simulink model "Simulink_ROS_Boat_Path_Follow_V2_5"  (R2025b)
settings: Solver=FixedStepAuto  StartTime=0.0  StopTime=2500  FixedStep=0.001  RelTol=1e-3
undefined symbols (not defined in the file): init_psi, init_x, init_y, path_x, path_y
libraries: ros2lib x6, slpidlib x2
settings Model: NumberOfSteps=10  Creator=Semih  LastModifiedBy=gehan
settings SolverCC: EnableFixedStepZeroCrossing=on

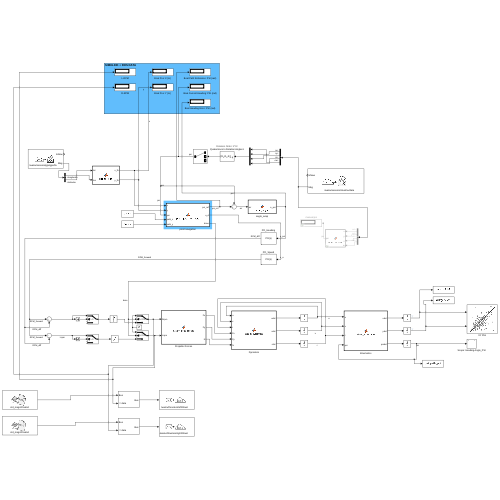
[thumbnail: Simulink's stored preview of the top-level diagram]
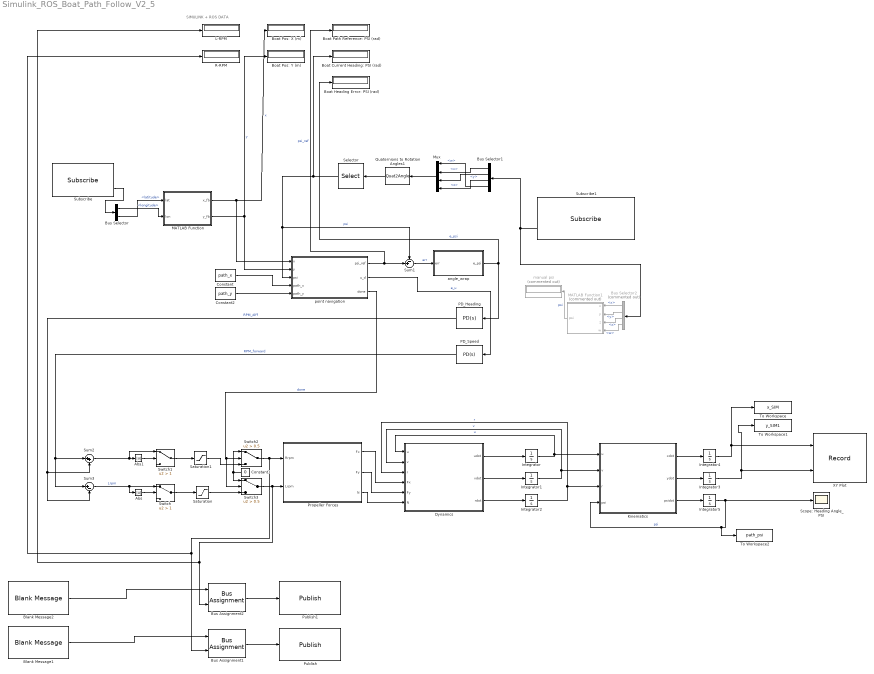
== system Simulink_ROS_Boat_Path_Follow_V2_5 ==
  note: SIMULINK + ROS DATA
  Abs : Abs  SaturateOnIntegerOverflow=off
  Abs1 : Abs  SaturateOnIntegerOverflow=off
  Blank Message1 : ros2lib/Blank Message  messageClass=Message  entityType=std_msgs/Float64  messageType=std_msgs/Float64  SampleTime=inf
  Blank Message2 : ros2lib/Blank Message  messageClass=Message  entityType=std_msgs/Float64  messageType=std_msgs/Float64  SampleTime=inf
  Boat Current Heading: PSI (rad) : Display
  Boat Heading Error: PSI (rad) : Display
  Boat Path Reference: PSI (rad) : Display
  Boat Pos: X (m) : Display
  Boat Pos: Y (m) : Display
  Bus Assignment1 : BusAssignment  AssignedSignals=data
  Bus Assignment2 : BusAssignment  AssignedSignals=data
  Bus Selector : BusSelector  OutputSignals=longitude,latitude
  Bus Selector1 : BusSelector  OutputSignals=orientation.x,orientation.y,orientation.z,orientation.w
  Bus Selector2 : BusSelector  Commented=on  OutputSignals=orientation.x,orientation.y,orientation.z,orientation.w
  Constant : Constant  Value=path_x
  Constant1 : Constant  Value=0
  Constant2 : Constant  Value=path_y
  Dynamics : MATLAB Function  TreatAsAtomicUnit=on
  Integrator : Integrator
  Integrator1 : Integrator
  Integrator2 : Integrator
  Integrator3 : Integrator  InitialCondition=init_y
  Integrator4 : Integrator  InitialCondition=init_x
  Integrator5 : Integrator  InitialCondition=init_psi
  Kinematics : MATLAB Function  TreatAsAtomicUnit=on
  L-RPM : Display
  MATLAB Function : MATLAB Function  TreatAsAtomicUnit=on
  MATLAB Function1 : MATLAB Function  Commented=on  TreatAsAtomicUnit=on
  Mux : Mux
  PD_Heading : slpidlib/PID Controller  Controller=PD  Form=Parallel  TimeDomain=Continuous-time  UseExternalTs=off  SampleTime=-1  IntegratorMethod=Forward Euler  FilterMethod=Forward Euler  ControllerParametersSource=internal  P=200  I=0  UseKiTs=off  D=5  UseExternalDerivativeSource=off  N=50  UseFilter=on  TunerSelectOption=Transfer Function Based (PID Tuner App)  InitialConditionSource=internal  InitialConditionForIntegrator=0  InitialConditionForFilter=0  DifferentiatorICPrevScaledInput=0  ExternalReset=none  TrackingMode=off  Kt=1  LimitOutput=off  SatLimitsSource=internal  UpperSaturationLimit=300  LowerSaturationLimit=-300  LinearizeAsGain=on  AntiWindupMode=back-calculation  Kb=1  LimitIntegrator=off  UpperIntegratorSaturationLimit=inf  LowerIntegratorSaturationLimit=-inf  POutMin=[]  POutMax=[]  IOutMin=[]  IOutMax=[]  DOutMin=[]  DOutMax=[]  NOutMin=[]  NOutMax=[]  SumOutMin=[]  SumOutMax=[]  SaturationOutMin=[]  SaturationOutMax=[]  PParamMin=[]  PParamMax=[]  IParamMin=[]  IParamMax=[]  DParamMin=[]  DParamMax=[]  NParamMin=[]  NParamMax=[]  KbParamMin=[]  KbParamMax=[]  KtParamMin=[]  KtParamMax=[]  KbOutMin=[]  KbOutMax=[]  KtOutMin=[]  KtOutMax=[]  IntegratorOutMin=[]  IntegratorOutMax=[]  FilterOutMin=[]  FilterOutMax=[]  SumI1OutMin=[]  SumI1OutMax=[]  SumI2OutMin=[]  SumI2OutMax=[]  SumI3OutMin=[]  SumI3OutMax=[]  SumI4OutMin=[]  SumI4OutMax=[]  SumDOutMin=[]  SumDOutMax=[]  DifferentiatorOutMin=[]  DifferentiatorOutMax=[]  FilterDiffOutCoefMin=[]  FilterDiffOutCoefMax=[]  ReciprocalOutMin=[]  ReciprocalOutMax=[]  SumDenOutMin=[]  SumDenOutMax=[]  SumNumOutMin=[]  SumNumOutMax=[]  DivideOutMin=[]  DivideOutMax=[]  UdiffTsProdOutMin=[]  UdiffTsProdOutMax=[]  NTsProdOutMin=[]  NTsProdOutMax=[]  UintegralTsProdOutMin=[]  UintegralTsProdOutMax=[]  UngainTsProdOutMin=[]  UngainTsProdOutMax=[]  ClampingZeroOutDataTypeStr=Inherit: Inherit via back propagation  ClampingZeroOutMin=[]  ClampingZeroOutMax=[]  FilterDenConstantOutDataTypeStr=Inherit: Inherit via back propagation  FilterDenConstantOutMin=[]  FilterDenConstantOutMax=[]  PCopyOutDataTypeStr=Inherit: Inherit via back propagation  PCopyOutMin=[]  PCopyOutMax=[]  NCopyOutDataTypeStr=Inherit: Inherit via back propagation  NCopyOutMin=[]  NCopyOutMax=[]  IntegratorContinuousStateAttributes=''  IntegratorStateMustResolveToSignalObject=off  IntegratorRTWStateStorageClass=Auto  FilterContinuousStateAttributes=''  FilterStateMustResolveToSignalObject=off  FilterRTWStateStorageClass=Auto  ParallelPVariant=InternalParameters  IdealPVariant=Disabled  IVariant=Disabled  DVariant=InternalParameters  IntegratorVariant=Disabled  SatVariant=Disabled  AWVariant=Disabled  PCopyVariant=Disabled  TRVariant=Disabled  FdbkBlocksVariant=Forward  IdealPFdbkVariant=Disabled  SatFdbkVariant=Disabled  DerivativeFilterVariant=ContFilter  NVariant=InternalParameters  NCopyVariant=Disabled  FilterICVariant=InternalICsFilter  IntegratorICVariant=Disabled  ExternalResetVariant=Disabled  TRSumVariant=Passthrough  SumFdbkVariant=Disabled  SumVariant=Sum_PD  TsampFilterVariant=InternalTs  TsampNgainVariant=Passthrough  TsampIntegralVariant=Disabled_SignalSpec  ExternalSaturationOutDataTypeStr=Inherit: Same as second input  DerivativeSourceVariant=ErrorSignal  PreIntVariant=InternalPreInt
  PD_Speed : slpidlib/PID Controller  Controller=PD  Form=Parallel  TimeDomain=Continuous-time  UseExternalTs=off  SampleTime=-1  IntegratorMethod=Forward Euler  FilterMethod=Forward Euler  ControllerParametersSource=internal  P=100  I=5  UseKiTs=off  D=5  UseExternalDerivativeSource=off  N=50  UseFilter=on  TunerSelectOption=Transfer Function Based (PID Tuner App)  InitialConditionSource=internal  InitialConditionForIntegrator=0  InitialConditionForFilter=0  DifferentiatorICPrevScaledInput=0  ExternalReset=none  TrackingMode=off  Kt=1  LimitOutput=off  SatLimitsSource=internal  UpperSaturationLimit=inf  LowerSaturationLimit=-inf  LinearizeAsGain=on  AntiWindupMode=none  Kb=1  LimitIntegrator=off  UpperIntegratorSaturationLimit=inf  LowerIntegratorSaturationLimit=-inf  POutMin=[]  POutMax=[]  IOutMin=[]  IOutMax=[]  DOutMin=[]  DOutMax=[]  NOutMin=[]  NOutMax=[]  SumOutMin=[]  SumOutMax=[]  SaturationOutMin=[]  SaturationOutMax=[]  PParamMin=[]  PParamMax=[]  IParamMin=[]  IParamMax=[]  DParamMin=[]  DParamMax=[]  NParamMin=[]  NParamMax=[]  KbParamMin=[]  KbParamMax=[]  KtParamMin=[]  KtParamMax=[]  KbOutMin=[]  KbOutMax=[]  KtOutMin=[]  KtOutMax=[]  IntegratorOutMin=[]  IntegratorOutMax=[]  FilterOutMin=[]  FilterOutMax=[]  SumI1OutMin=[]  SumI1OutMax=[]  SumI2OutMin=[]  SumI2OutMax=[]  SumI3OutMin=[]  SumI3OutMax=[]  SumI4OutMin=[]  SumI4OutMax=[]  SumDOutMin=[]  SumDOutMax=[]  DifferentiatorOutMin=[]  DifferentiatorOutMax=[]  FilterDiffOutCoefMin=[]  FilterDiffOutCoefMax=[]  ReciprocalOutMin=[]  ReciprocalOutMax=[]  SumDenOutMin=[]  SumDenOutMax=[]  SumNumOutMin=[]  SumNumOutMax=[]  DivideOutMin=[]  DivideOutMax=[]  UdiffTsProdOutMin=[]  UdiffTsProdOutMax=[]  NTsProdOutMin=[]  NTsProdOutMax=[]  UintegralTsProdOutMin=[]  UintegralTsProdOutMax=[]  UngainTsProdOutMin=[]  UngainTsProdOutMax=[]  ClampingZeroOutDataTypeStr=Inherit: Inherit via back propagation  ClampingZeroOutMin=[]  ClampingZeroOutMax=[]  FilterDenConstantOutDataTypeStr=Inherit: Inherit via back propagation  FilterDenConstantOutMin=[]  FilterDenConstantOutMax=[]  PCopyOutDataTypeStr=Inherit: Inherit via back propagation  PCopyOutMin=[]  PCopyOutMax=[]  NCopyOutDataTypeStr=Inherit: Inherit via back propagation  NCopyOutMin=[]  NCopyOutMax=[]  IntegratorContinuousStateAttributes=''  IntegratorStateMustResolveToSignalObject=off  IntegratorRTWStateStorageClass=Auto  FilterContinuousStateAttributes=''  FilterStateMustResolveToSignalObject=off  FilterRTWStateStorageClass=Auto  ParallelPVariant=InternalParameters  IdealPVariant=Disabled  IVariant=Disabled  DVariant=InternalParameters  IntegratorVariant=Disabled  SatVariant=Disabled  AWVariant=Disabled  PCopyVariant=Disabled  TRVariant=Disabled  FdbkBlocksVariant=Forward  IdealPFdbkVariant=Disabled  SatFdbkVariant=Disabled  DerivativeFilterVariant=ContFilter  NVariant=InternalParameters  NCopyVariant=Disabled  FilterICVariant=InternalICsFilter  IntegratorICVariant=Disabled  ExternalResetVariant=Disabled  TRSumVariant=Passthrough  SumFdbkVariant=Disabled  SumVariant=Sum_PD  TsampFilterVariant=InternalTs  TsampNgainVariant=Passthrough  TsampIntegralVariant=Disabled_SignalSpec  ExternalSaturationOutDataTypeStr=Inherit: Same as second input  DerivativeSourceVariant=ErrorSignal  PreIntVariant=InternalPreInt
  Propeller Forces : MATLAB Function  TreatAsAtomicUnit=on
  Publish : ros2lib/Publish  topicSource=Specify your own  topic=/wamv/thrusters/right/thrust  messageType=std_msgs/Float64  QOSHistory=Keep last  QOSDepth=10  QOSReliability=Reliable  QOSDurability=Volatile  QOSDeadline=Inf  QOSLifespan=Inf  QOSLiveliness=Automatic  QOSLeaseDuration=Inf  QOSAvoidROSNamespaceConventions=off
  Publish1 : ros2lib/Publish  topicSource=Specify your own  topic=/wamv/thrusters/left/thrust  messageType=std_msgs/Float64  QOSHistory=Keep last  QOSDepth=10  QOSReliability=Reliable  QOSDurability=Volatile  QOSDeadline=Inf  QOSLifespan=Inf  QOSLiveliness=Automatic  QOSLeaseDuration=Inf  QOSAvoidROSNamespaceConventions=off
  Quaternions to Rotation Angles1 : Quat2Angle
      settings: AttributesFormatString=Rotation Order: %<rotationOrder>
  R-RPM : Display
  Saturation : Saturate  UpperLimit=1000  LowerLimit=0
  Saturation1 : Saturate  UpperLimit=1000  LowerLimit=0
  Scope: Heading Angle_PSI : Scope
      settings: ActiveDisplayYMinimum=-6.15148375375635  ActiveDisplayYMaximum=4.7778710179272776
  Selector : Selector  InputPortWidth=3  IndexOptions=Index vector (dialog)  Indices=1  OutputSizes=1
  Subscribe : ros2lib/Subscribe  topicSource=Specify your own  topic=/wamv/sensors/gps/gps/fix  messageType=sensor_msgs/NavSatFix  sampleTime=-1  QOSHistory=Keep last  QOSDepth=10  QOSReliability=Reliable  QOSDurability=Volatile  QOSDeadline=Inf  QOSLifespan=Inf  QOSLiveliness=Automatic  QOSLeaseDuration=Inf  QOSAvoidROSNamespaceConventions=off
  Subscribe1 : ros2lib/Subscribe  topicSource=Specify your own  topic=/wamv/sensors/imu/imu/data  messageType=sensor_msgs/Imu  sampleTime=-1  QOSHistory=Keep last  QOSDepth=10  QOSReliability=Reliable  QOSDurability=Volatile  QOSDeadline=Inf  QOSLifespan=Inf  QOSLiveliness=Automatic  QOSLeaseDuration=Inf  QOSAvoidROSNamespaceConventions=off
  Sum1 : Sum  Inputs=-+|
  Sum2 : Sum  Inputs=|++
  Sum3 : Sum  Inputs=|+-
  Switch : Switch  Criteria=u2 > Threshold  Threshold=1  SaturateOnIntegerOverflow=off  InputSameDT=off
  Switch1 : Switch  Criteria=u2 > Threshold  Threshold=1  SaturateOnIntegerOverflow=off  InputSameDT=off
  Switch2 : Switch  Criteria=u2 > Threshold  Threshold=0.5  SaturateOnIntegerOverflow=off  InputSameDT=off
  Switch3 : Switch  Criteria=u2 > Threshold  Threshold=0.5  SaturateOnIntegerOverflow=off  InputSameDT=off
  To Workspace : ToWorkspace  VariableName=x_SIM  SaveFormat=Timeseries  SampleTime=-1
  To Workspace1 : ToWorkspace  VariableName=y_SIM1  SaveFormat=Timeseries  SampleTime=-1
  To Workspace2 : ToWorkspace  VariableName=path_psi  SaveFormat=Timeseries  SampleTime=-1
  XY Plot : Record  NumPorts=2.0  FileSettingsInternal="{\"entries\":[{\"content\":{\"excelSettings\":{\"content\":{},\"type\":\"Streamout.ExcelSettings\"},\"parquetSettings\":{\"content\":{},\"type\":\"Streamout.ParquetSettings\"}},\"type\":\"Streamout.FileSettingStorage\",\"uuid\":\"\"}],\"packageUris\":[\"http:\\/\\/schema.mathworks.com\\/mf0\\/streamout_blocks\\/R2020a\"],\"version\":\"1.0\"}"  FrameSettings=[0, 0]  Layout=[1 1]  SignalsInternal="{\"entries\":[{\"content\":{\"signals\":[{\"content\":{\"blockPath\":[],\"dimensions\":[1],\"domain\":\"\",\"lineColor\":\"#fe330a\",\"lineWidth\":2,\"port\":1,\"signalID\":1,\"signalName\":\"Integrator4\"},\"type\":\"RecordBlkView.Signal\",\"uuid\":\"\"},{\"content\":{\"blockPath\":[],\"dimensions\":[1],\"domain\":\"\",\"lineColor\":\"#139fff\",\"plots\":[ 1 ],\"port\":2,\"signalID\":2,\"signalName\":\"Integrator3\"},\"type\":\"RecordBlkView.Signal\",\"uuid\":\"\"}]},\"type\":\"RecordBlkView.InputSignals\",\"uuid\":\"\"}],\"packageUris\":[\"http:\\/\\/schema.mathworks.com\\/mf0\\/streamout_blocks\\/R2020a\"],\"version\":\"1.0\"}"  VisualizationBindings="{\"xyplotplugin\":{\"info\":[{\"series\":[{\"bindingParametersList\":[{\"parameter\":\"Y-Axis\",\"signalID\":2,\"signalName\":\"Integrator3\"}],\"seriesID\":0}],\"subplotID\":1}]}}"  CompatibilityTag=XY
  angle_wrap : MATLAB Function  TreatAsAtomicUnit=on
  manual psi : Display  Commented=on
  point navigation : MATLAB Function  TreatAsAtomicUnit=on
  wires:
  Dynamics/1(udot) -> Integrator/1
  Dynamics/2(vdot) -> Integrator1/1
  Dynamics/3(rdot) -> Integrator2/1
  Integrator/1 -> Dynamics/1(u), Kinematics/1(u)  "u"
  Integrator1/1 -> Dynamics/2(v), Kinematics/2(v)  "v"
  Integrator2/1 -> Dynamics/3(r), Kinematics/3(r)  "r"
  Kinematics/1(xdot) -> Integrator4/1
  Kinematics/2(ydot) -> Integrator3/1
  Kinematics/3(psidot) -> Integrator5/1
  Integrator4/1 -> To Workspace/1, XY Plot/1
  Propeller Forces/1(Fx) -> Dynamics/4(Fx)
  Propeller Forces/2(Fy) -> Dynamics/5(Fy)
  Propeller Forces/3(N) -> Dynamics/6(N)
  Integrator3/1 -> To Workspace1/1, XY Plot/2
  Integrator5/1 -> To Workspace2/1, Kinematics/4(psi), Scope: Heading Angle_PSI/1  "psi"
  PD_Heading/1 -> Sum3/2, Sum2/2  "RPM_diff"
  angle_wrap/1(e_psi) -> PD_Heading/1, Boat Heading Error: PSI (rad)/1  "e_psi"
  point navigation/2(u_d) -> PD_Speed/1  "e_u"
  PD_Speed/1 -> Sum2/1, Sum3/1  "RPM_forward"
  Sum2/1 -> Switch1/1, Abs1/1
  Sum3/1 -> Abs/1, Switch/1  "Lrpm"
  point navigation/1(psi_ref) -> Boat Path Reference: PSI (rad)/1, Sum1/2  "psi_ref"
  Sum1/1 -> angle_wrap/1(err)  "err"
  Constant/1 -> point navigation/4(path_x)
  Constant2/1 -> point navigation/5(path_y)
  Blank Message1/1 -> Bus Assignment1/1
  Bus Assignment1/1 -> Publish/1
  Bus Assignment2/1 -> Publish1/1
  Blank Message2/1 -> Bus Assignment2/1
  Subscribe/2 -> Bus Selector/1
  Bus Selector/1 -> MATLAB Function/2(lon)  "<longitude>"
  Bus Selector/2 -> MATLAB Function/1(lat)  "<latitude>"
  MATLAB Function/1(x_fb) -> point navigation/1(x), Boat Pos: X (m)/1  "x"
  MATLAB Function/2(y_fb) -> point navigation/2(y), Boat Pos: Y (m)/1  "y"
  Selector/1 -> Sum1/1, point navigation/3(psi), Boat Current Heading: PSI (rad)/1  "psi"
  Subscribe1/2 -> Bus Selector1/1, Bus Selector2/1
  Bus Selector1/1 -> Mux/2  "<x>"
  Bus Selector1/2 -> Mux/3  "<y>"
  Bus Selector1/3 -> Mux/4  "<z>"
  Bus Selector1/4 -> Mux/1  "<w>"
  Mux/1 -> Quaternions to Rotation Angles1/1
  Quaternions to Rotation Angles1/1 -> Selector/1
  Bus Selector2/1 -> MATLAB Function1/1(x)  "<x>"
  Bus Selector2/2 -> MATLAB Function1/2(y)  "<y>"
  Bus Selector2/3 -> MATLAB Function1/3(z)  "<z>"
  Bus Selector2/4 -> MATLAB Function1/4(w)  "<w>"
  MATLAB Function1/1(psi) -> manual psi/1  "psi"
  Saturation1/1 -> Switch2/3
  Saturation/1 -> Switch3/3
  Switch/1 -> Saturation/1
  Abs/1 -> Switch/2
  Abs1/1 -> Switch1/2
  Switch1/1 -> Saturation1/1
  Switch2/1 -> Propeller Forces/1(Rrpm), R-RPM/1, Bus Assignment1/2
  point navigation/3(done) -> Switch3/2, Switch2/2  "done"
  Switch3/1 -> L-RPM/1, Bus Assignment2/2, Propeller Forces/2(Lrpm)
  Constant1/1 -> Switch2/1, Switch3/1

== matlab function Simulink_ROS_Boat_Path_Follow_V2_5/Dynamics ==
  data: u input; udot output; v input; r input; Fx input; Fy input; N input; vdot output; rdot output
function [udot, vdot, rdot] = catam_dynamics(u, v, r, Fx, Fy, N)
%% CATAM_DYNAMICS - Equations of Motion (Eqn-2)
%  Calculates accelerations in the body-fixed frame.
%
%  Inputs:
%    u, v, r    : Surge, Sway, Yaw velocities [m/s, m/s, rad/s]
%    Fx, Fy, N  : External Forces and Moment [N, N, Nm]
%
%  Outputs:
%    udot, vdot, rdot : Accelerations [m/s^2, m/s^2, rad/s^2]

    %% ---- PARAMETERS ----
    % 1. Mass and Inertia Properties
    m   = 100;        % Mass of catamaran [kg] ; Reserach Paper m = 225
    Izz = 100;     % Moment of inertia about Z-axis [kg m^2]; Reserach Paper Izz = 144.75

    % 2. Added Mass (Eq 11)
    m11 = 15.82;      % Added mass in surge [kg]
    m22 = 118.36;     % Added mass in sway [kg]
    m66 = 31.36;      % Added rotational inertia [kg m^2]

    % 3. Hydrodynamic Resistance Coefficients
    d11 = 171.2;      % Longitudinal resistance [kg/s]
    d22 = 342.4;      % Lateral resistance [kg/s] (Assumed 2*d11)
    d33 = 557;        % Rotational resistance [kg m^2/s]

    %% ---- DYNAMICS EQUATIONS (Eqn 2) ----

    % Surge acceleration (u-dot)
    % Equation 2a: (m + m11)*udot = Fx - m*v*r - d11*u
    udot = (Fx - m*v*r - d11*u) / (m + m11);

    % Sway acceleration (v-dot)
    % Equation 2b: (m + m22)*vdot = Fy + m*u*r - d22*v
    vdot = (Fy + m*u*r - d22*v) / (m + m22);

    % Yaw acceleration (r-dot)
    % Equation 2c: (Izz + m66)*rdot = N - d33*r
    rdot = (N - d33*r) / (Izz + m66);

end

== matlab function Simulink_ROS_Boat_Path_Follow_V2_5/Propeller Forces ==
  data: Rrpm input; Lrpm input; Fx output; Fy output; N output
function [Fx, Fy, N] = catam_prop_forces(Rrpm, Lrpm)

%% Eqn-3 - PROP_FORCES Function

%% ---- CONSTANTS ----
dNP = 0.25;          % turning moment correction factor
d   = 0.405;         % half-hull spacing (Halfwidth) [m]
rho = 1000;          % water density [kg/m^3]
dPL = 0.18;          % propeller diameter left [m]
dPR = 0.18;          % propeller diameter right [m]
a_p = 0.2205;        % unified thrust coefficient @ rho = 1000 kg/m^3
tp  = 0.25;          % thrust deduction factor

%% RPM to RPS
nL = Lrpm/60;
nR = Rrpm/60;

%% Properller Thrust - Eqn 4
FL = a_p * rho * nL^2 * dPL^4;
FR = a_p * rho * nR^2 * dPR^4;

%% Forces and moment
Fx = (1 - tp) * (FL + FR);
Fy = 0;
N  = (1 + dNP) * (FR - FL) * d;

end

== matlab function Simulink_ROS_Boat_Path_Follow_V2_5/Kinematics ==
  data: u input; xdot output; v input; r input; psi input; ydot output; psidot output
function [xdot, ydot, psidot] = catam_kinematics(u,v,r,psi)
%% CATAMARAN_KINEMATICS Summary of this function goes here - Eqn-1

%% Heading rate
psidot = r;

%% Earth-fixed velocities
xdot = u*cos(psi) - v*sin(psi);
ydot = u*sin(psi) + v*cos(psi);

end

== matlab function Simulink_ROS_Boat_Path_Follow_V2_5/angle_wrap ==
  data: err input; e_psi output
function e_psi = wrap_angle(err)
e_psi = wrapToPi(err);
end

== matlab function Simulink_ROS_Boat_Path_Follow_V2_5/MATLAB Function ==
  data: x_fb output; y_fb output; lat input; lon input
function [x_fb, y_fb] = gps_to_local(lat, lon)
    % Persistent variables to remember the starting location
    persistent lat0 lon0 has_origin
    
    % Initialize origin at the very first step
    if isempty(has_origin)
        lat0 = lat;
        lon0 = lon;
        has_origin = true;
    end
    
    % Calculate distance (in meters) from the starting point
    origin = [lat0, lon0, 0];
    [x_rel, y_rel, ~] = latlon2local(lat, lon, 0, origin);
    % x_rel = Distance East from start
    % y_rel = Distance North from start
    
    % Map East to X, North to Y
    % Boat starts at Gazebo X = -532.0, Y = 161.998
    x_fb = x_rel - 532.0;   
    y_fb = y_rel + 161.996; 
end

== matlab function Simulink_ROS_Boat_Path_Follow_V2_5/MATLAB Function1 ==
  data: x input; psi output; y input; z input; w input
function psi = quat_to_yaw(x, y, z, w)
    % Calculate Yaw (psi) from Quaternion
    siny_cosp = 2 * (w * z + x * y);
    cosy_cosp = 1 - 2 * (y * y + z * z);
    psi = atan2(siny_cosp, cosy_cosp);

    %psi = 0;
end

== matlab function Simulink_ROS_Boat_Path_Follow_V2_5/point navigation ==
  settings: updateMethod=DISCRETE
  data: psi_ref output; x input; y input; u_d output; psi input; path_x input; path_y input; done output
function [psi_ref, u_d, done] = path_guidance_theta(x, y, psi, path_x, path_y)
    % =====================================================================
    % PATH_GUIDANCE_THETA
    % 
    % Implements Adaptive Pure Pursuit Guidance with the following features:
    % 1. Quadratic Line-Circle Intersection: For smooth "Rabbit" tracking.
    % 2. Square-Root Deceleration: Drops u_d (forward) aggressively to force RPM reduction.
    % 3. Heading Latch: Freezes psi_ref prevent stop-point jitter when stop point is closer.
    % 4. Termination: Signals to motor cutoff
    % =====================================================================

    % 1. INITIALIZATION & PERSISTENT MEMORY
    persistent parking_completed last_good_psi
    if isempty(parking_completed)
        parking_completed = false;
        last_good_psi = psi; % Initialize with current boat heading
    end
    
    % 2. CONTROL PARAMETERS
    u_max        = 2.0;    % Maximum cruise speed [m/s]
    u_min        = 0.1;    % Minimum crawl speed floor [m/s]
    look_dist    = 8.0;    % Nominal lookahead distance [m]
    slow_radius  = 12.0;   % Zone to begin deceleration  
    stop_radius  = 5.0;    % Radius to trigger mission completion [m]
    latch_radius = 3.5;    % Radius to freeze heading calculations to avoid fluctuation in the end (Jitter)

    % 3. DISTANCE CALCULATIONS
    % Explicitly calculate distance to the absolute final waypoint
    target_x = path_x(end);
    target_y = path_y(end);
    dist_end = hypot(target_x - x, target_y - y);
    
    % Find the closest point index on the path for the Rabbit Search
    dx_all = path_x - x;
    dy_all = path_y - y;
    [~, k] = min(dx_all.^2 + dy_all.^2); 
    
    % 4. ADAPTIVE LOOKAHEAD RADIUS (R)
    if dist_end > 5.0
        R = look_dist; % Radius of the Rabbit Circle
    else
        R = max(1.0, dist_end * 0.8); % Radius of the Rabbit Circle is Reduced - Approaching Target
    end
    
    % 5. FIND INTERSECTION (THE RABBIT)
    rabbit_x = target_x;
    rabbit_y = target_y;
    
    for i = k : length(path_x)-1
        p1x = path_x(i) - x;   p1y = path_y(i) - y;
        p2x = path_x(i+1) - x; p2y = path_y(i+1) - y;
        d2 = hypot(p2x, p2y);
        
        if d2 > R
            dx_seg = p2x - p1x; 
            dy_seg = p2y - p1y;
            a = dx_seg^2 + dy_seg^2;
            b = 2 * (p1x * dx_seg + p1y * dy_seg);
            c = (p1x^2 + p1y^2) - R^2;
            delta = b^2 - 4*a*c;
            
            if delta >= 0
                t = (-b + sqrt(delta)) / (2*a);
                t = max(0, min(1, t)); 
                rabbit_x = path_x(i) + t * (path_x(i+1) - path_x(i));
                rabbit_y = path_y(i) + t * (path_y(i+1) - path_y(i));
                break; 
            end
        end
    end

    % 6. HEADING LOGIC (Jitter Prevention)
    if dist_end > latch_radius && ~parking_completed
        psi_ref = atan2(rabbit_y - y, rabbit_x - x);
        last_good_psi = psi_ref; % When Far From Target, Update the PSI with arctan
    else
        psi_ref = last_good_psi; % When Closer To Target, Not Update the PSI with arctan
    end
    
    % 7. SPEED PROFILE (Slowing Down near Target)
    if dist_end < slow_radius
        norm_dist = (dist_end - stop_radius) / (slow_radius - stop_radius); %Progress Bar Logic to Map 0 to 1
        norm_dist = max(0, min(1, norm_dist));
        u_d = u_min + (u_max - u_min) * sqrt(norm_dist);
    else
        u_d = u_max;
    end
    
    % Turn-Then-Go (When Heading Error is Larger, Slow Down Boat) 
    e_theta = wrapToPi(psi_ref - psi);
    u_d = u_d * max(0, cos(e_theta));

    % 8. STOP LOGIC (TERMINATION MOTORS)
     if (dist_end <= stop_radius) || parking_completed
        u_d = 0;             
        done = true;         
        parking_completed = true;
    else
        done = false;
    end
end
